simulink model "Parsim_for_3level"  (R2024b)
settings: Solver=FixedStepDiscrete  StartTime=0.0  StopTime=1  FixedStep=Ts  RelTol=1e-3
PreLoadFcn:
  | Net_improve_init;L=Lac_MV;Ts=20e-6;Tctrl=Ts;Rac_MV=1;
PostLoadFcn:
  | Net_improve_init;L=Lac_MV;Ts=20e-6;Tctrl=Ts;Rac_MV=1;
InitFcn:
  | Net_improve_init;L=Lac_MV;Ts=20e-6;Tctrl=Ts;Rac_MV=1;
undefined symbols (not defined in the file or in its folder): C1, dend, DiscIntNeverNeededParam, fs, Lac_MV, numd, Pref, R1, Vac_peak_MV, Vdc
libraries: spsIGBTDiodeLib x12, powerlib_extras x10, spsControlledVoltageSourceLib x8, spsCurrentMeasurementLib x6, spsSeriesRLCBranchLib x6, spsVoltageMeasurementLib x6, spsThreePhaseVIMeasurementLib x4, spsGroundLib x4, spsIdealSwitchLib x2, spsPower3phInstantaneousLib x2, simulink x2, spsThreePhaseSeriesRLCBranchLib x2
(part 2 of 2)

== system Parsim_for_3level/Rec_VQcontrol1/pqctrl/dq ctlr/measure ==
  note: this is to validate Rxpu and Lxpu which make PI(error) almost zero,
      | i.e. the delay is properly set
      |
      | or to calculate Rxpu and Lxpu which make PI(error) zero
      | when input are in steady state
      |
      | when change the P,Q ref,
      | the results should be same if delay is properly cancelled
  A=X-V : Inport
  Idqref : Inport  Port=2
  Display1 : Display
      settings: Decimation=200
  Fcn7 : Fcn  Expr=(u[2] *u[3]-u[1]*u[4])/(u[3]^2+u[4]^2)
  Fcn8 : Fcn  Expr=(u[1] *u[3]+u[2]*u[4])/(u[3]^2+u[4]^2)
  Mux3 : Mux  Inputs=2
  Mux4 : Mux  Inputs=2
  wires:
  Mux3/1 -> Fcn8/1, Fcn7/1
  Fcn8/1 -> Mux4/1  "Rxpu"
  Fcn7/1 -> Mux4/2  "Lxpu"
  A=X-V/1 -> Mux3/1
  Idqref/1 -> Mux3/2
  Mux4/1 -> Display1/1

== system Parsim_for_3level/Rec_VQcontrol3/Vdc ctrl/Vdc_ctrler1/PI_d2 ==
  note: Discrete PID Controller
  note: Pierre Giroux, Gilbert Sybille
      | Power System Simulation Laboratory
      | IREQ, Hydro-Quebc
  Error : Inport  SampleTime=Ts
  Discrete-Time Integrator : DiscreteIntegrator  InitialCondition=Init  SampleTime=Ts  LimitOutput=on  UpperSaturationLimit=UpperLimit  LowerSaturationLimit=LowerLimit  ICPrevOutput=DiscIntNeverNeededParam  ICPrevScaledInput=DiscIntNeverNeededParam
  Kp4 : Gain  Gain=Kp  SaturateOnIntegerOverflow=on  SampleTime=Ts  OutDataTypeStr=Inherit: Same as input  ParamDataTypeStr=Inherit: Same as input
  Kp5 : Gain  Gain=Ki  SaturateOnIntegerOverflow=on  SampleTime=Ts  OutDataTypeStr=Inherit: Same as input  ParamDataTypeStr=Inherit: Same as input
  Saturation2 : Saturate  UpperLimit=UpperLimit  LowerLimit=LowerLimit  SampleTime=Ts
  Sum6 : Sum  InputSameDT=on  SaturateOnIntegerOverflow=on  SampleTime=Ts  OutDataTypeStr=Inherit: Same as first input
  Zero-Order Hold : ZeroOrderHold  SampleTime=Ts
  Out : Outport  SampleTime=Ts  InitialOutput=0  VectorParamsAs1DForOutWhenUnconnected=off
  wires:
  Zero-Order Hold/1 -> Sum6/1  "prop"
  Saturation2/1 -> Out/1
  Discrete-Time Integrator/1 -> Sum6/2  "int"
  Kp4/1 -> Zero-Order Hold/1
  Kp5/1 -> Discrete-Time Integrator/1
  Sum6/1 -> Saturation2/1
  Error/1 -> Kp5/1, Kp4/1

== system Parsim_for_3level/Rec_VQcontrol3/pqctrl/dq ctlr/Subsystem1 ==
  Vdq2 : Inport
  PQref : Inport  Port=2
  Fcn7 : Fcn  Expr=(u[1] *u[4]+u[2]*u[5])/u[3]
  Fcn8 : Fcn  Expr=(u[2] *u[4]-u[1]*u[5])/u[3]
  Fcn9 : Fcn  Expr=(u[1] ^2+u[2]^2)
  Mux3 : Mux  Inputs=[2 1 2]
  Mux4 : Mux  Inputs=2
  Saturation : Saturate  UpperLimit=inf  LowerLimit=0.01
  Saturation1 : Saturate  UpperLimit=1.5  LowerLimit=-1.5
  Idqref : Outport  VectorParamsAs1DForOutWhenUnconnected=off
  wires:
  Saturation1/1 -> Idqref/1
  Vdq2/1 -> Fcn9/1, Mux3/1
  Mux3/1 -> Fcn8/1, Fcn7/1
  Fcn9/1 -> Saturation/1
  Fcn7/1 -> Mux4/1
  Fcn8/1 -> Mux4/2
  Mux4/1 -> Saturation1/1  "Idqref"
  PQref/1 -> Mux3/3
  Saturation/1 -> Mux3/2

== system Parsim_for_3level/Rec_VQcontrol3/pqctrl/dq ctlr/Vdqref ==
  Vdq2 : Inport
  Idqref : Inport  Port=2
  Display : Display
      settings: Decimation=50
  Fcn7 : Fcn  Expr=(u[2] +u[4]*u[5]+u[3]*u[6])
  Fcn8 : Fcn  Expr=(u[1] +u[3]*u[5]-u[4]*u[6])
  Lxpu : Constant  Value=Lxpu
  Mux3 : Mux
  Mux4 : Mux  Inputs=2
  Rxpu : Constant  Value=Rxpu
  Vdqrefss : Outport  VectorParamsAs1DForOutWhenUnconnected=off
  wires:
  Lxpu/1 -> Mux3/4
  Rxpu/1 -> Mux3/3
  Mux3/1 -> Display/1, Fcn8/1, Fcn7/1
  Fcn8/1 -> Mux4/1  "Vdref"
  Fcn7/1 -> Mux4/2  "Vqref"
  Vdq2/1 -> Mux3/1
  Idqref/1 -> Mux3/2
  Mux4/1 -> Vdqrefss/1

== system Parsim_for_3level/Rec_VQcontrol3/pqctrl/dq ctlr/abc_dq ==
  abc : Inport
  theta : Inport  Port=2
  Mux2 : Mux  Inputs=2
  Selector3 : Selector  InputPortWidth=3  IndexOptions=Index vector (dialog)  Indices=[1 2]  OutputSizes=1
  Trigonometric Function2 : Trigonometry
  Trigonometric Function3 : Trigonometry  Operator=cos
  abc/dq1 : powerlib_extras/Measurements/abc_to_dq0 Transformation
  dq : Outport  VectorParamsAs1DForOutWhenUnconnected=off
  wires:
  abc/1 -> abc/dq1/1
  Selector3/1 -> dq/1
  abc/dq1/1 -> Selector3/1
  Mux2/1 -> abc/dq1/2
  theta/1 -> Trigonometric Function3/1, Trigonometric Function2/1
  Trigonometric Function2/1 -> Mux2/1
  Trigonometric Function3/1 -> Mux2/2

== system Parsim_for_3level/Rec_VQcontrol3/pqctrl/dq ctlr/abc_dq1 ==
  abc : Inport
  theta : Inport  Port=2
  Mux2 : Mux  Inputs=2
  Selector3 : Selector  InputPortWidth=3  IndexOptions=Index vector (dialog)  Indices=[1 2]  OutputSizes=1
  Trigonometric Function2 : Trigonometry
  Trigonometric Function3 : Trigonometry  Operator=cos
  abc/dq1 : powerlib_extras/Measurements/abc_to_dq0 Transformation
  dq : Outport  VectorParamsAs1DForOutWhenUnconnected=off
  wires:
  Trigonometric Function3/1 -> Mux2/2
  Trigonometric Function2/1 -> Mux2/1
  theta/1 -> Trigonometric Function2/1, Trigonometric Function3/1
  Mux2/1 -> abc/dq1/2
  abc/dq1/1 -> Selector3/1
  Selector3/1 -> dq/1
  abc/1 -> abc/dq1/1

== system Parsim_for_3level/Rec_VQcontrol3/pqctrl/dq ctlr/measure ==
  note: this is to validate Rxpu and Lxpu which make PI(error) almost zero,
      | i.e. the delay is properly set
      |
      | or to calculate Rxpu and Lxpu which make PI(error) zero
      | when input are in steady state
      |
      | when change the P,Q ref,
      | the results should be same if delay is properly cancelled
  A=X-V : Inport
  Idqref : Inport  Port=2
  Display1 : Display
      settings: Decimation=200
  Fcn7 : Fcn  Expr=(u[2] *u[3]-u[1]*u[4])/(u[3]^2+u[4]^2)
  Fcn8 : Fcn  Expr=(u[1] *u[3]+u[2]*u[4])/(u[3]^2+u[4]^2)
  Mux3 : Mux  Inputs=2
  Mux4 : Mux  Inputs=2
  wires:
  Mux3/1 -> Fcn8/1, Fcn7/1
  Fcn8/1 -> Mux4/1  "Rxpu"
  Fcn7/1 -> Mux4/2  "Lxpu"
  A=X-V/1 -> Mux3/1
  Idqref/1 -> Mux3/2
  Mux4/1 -> Display1/1
